simulink model "Pruning_observer_inexact"  (R2019b)
settings: Solver=VariableStepAuto  StartTime=0.0  StopTime=20  RelTol=1e-3
values from neighbouring files (symbols this model uses):
  d = 0.1    [Dynamicfcn.m]    (also in Run_this_file_for_DDWMR_model.m; gps.m)
  eta = 0.8    [Run_this_file_for_DDWMR_model.m]
  I = 0.05    [Dynamicfcn.m]    (also in Run_this_file_for_DDWMR_model.m = 0.26903125)
  L = 0.235/2    (= 0.1175)    [Dynamicfcn.m]    (also in Run_this_file_for_DDWMR_model.m; encoder.m)
  m = 10    [Dynamicfcn.m]    (also in Run_this_file_for_DDWMR_model.m = 15)
  q_initial = [theta_0;x_0;y_0]    [Run_this_file_for_DDWMR_model.m]
  r = 0.05    [Dynamicfcn.m]    (also in Run_this_file_for_DDWMR_model.m; encoder.m; robustness_support.m = temp_r(N+1:-1:1))
  R = 1e-3    (= 0.001)    [Run_this_file_for_DDWMR_model.m]
  rp = 0.6    [Run_this_file_for_DDWMR_model.m]
  s = 0.5    [Run_this_file_for_DDWMR_model.m]    (also in robustness_support.m = -(1-p)./p)
  Ts = 0.01    [Dynamicfcn.m]    (also in Run_this_file_for_DDWMR_model.m; gps.m = 0.001)
  V_initial = [v_0;w_0]    [Run_this_file_for_DDWMR_model.m]
libraries: simulink x3, sharedTrackingLibrary x1
settings Model: Creator=yu zheng  LastModifiedBy=yu zheng
settings DataIOCC: ReturnWorkspaceOutputsName=out_pruning

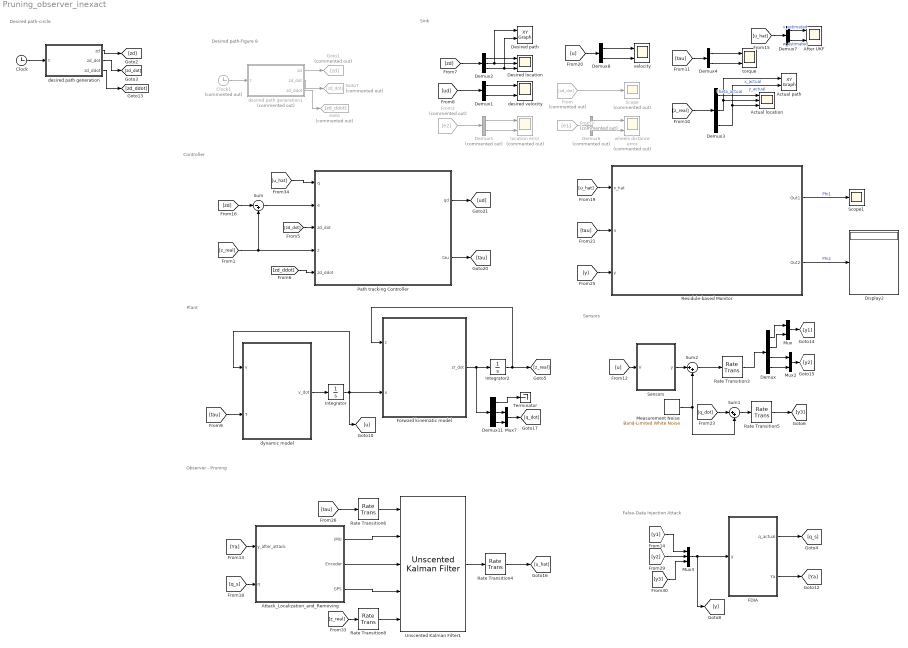
== system Pruning_observer_inexact ==
  note: Sink
  note: Controller
  note: Observer - Pruning
  note: Sensors
  note: Plant
  note: False-Data Injection Attack
  note: Desired path-circle
  note: Desired path-figure 8
  Actual location : Scope  NumInputPorts=3
  Actual path : simulink/Sinks/XY Graph  xmin=-2  xmax=2  ymin=-2  ymax=2  st=-1
  After UKF : Scope  NumInputPorts=2
  Attack_Localization_and_Removing : Subsystem
  Clock : Clock
  Clock1 : Clock  Commented=on
  Demux : Demux
  Demux{1,4,7..8} (4 alike) : Demux  Outputs=2
  Demux11 : Demux  Outputs=3
  Demux2 : Demux  Outputs=3
  Demux3 : Demux  Outputs=3
  Demux5 : Demux  Commented=on  Outputs=2
  Demux6 : Demux  Commented=on  Outputs=2
  Desired location : Scope  NumInputPorts=3
  "Desired path " : simulink/Sinks/XY Graph  xmin=-2  xmax=2  ymin=-2  ymax=2  st=-1
  Display2 : Display
  FDIA : MATLAB Function  TreatAsAtomicUnit=on
  Forward kinematic model : MATLAB Function  TreatAsAtomicUnit=on
  From : From  Commented=on  GotoTag=ud_dot
  From2 : From  Commented=on  GotoTag=e2
  From3 : From  Commented=on  GotoTag=e1
  Goto : Goto  Commented=on  GotoTag=zd_ddot
  Goto1 : Goto  Commented=on  GotoTag=zd
  Goto7 : Goto  Commented=on  GotoTag=zd_dot
  Integrator : Integrator  InitialCondition=V_initial
  Integrator2 : Integrator  InitialCondition=q_initial
  Measurement Noise : simulink/Sources/Band-Limited White Noise  Cov=R*Ts  Ts=Ts  seed=[23341]
  Mux : Mux  Inputs=2
  Mux2 : Mux  Inputs=2
  Mux3 : Mux  Inputs=3
  Mux7 : Mux  Inputs=2
  Path tracking Controller : MATLAB Function  TreatAsAtomicUnit=on
  Rate Transition3 : RateTransition  InitialCondition=[0 0 0 0]  OutPortSampleTime=Ts
  Rate Transition4 : RateTransition  Integrity=off  InitialCondition=1.6  OutPortSampleTime=0
  Rate Transition5 : RateTransition  InitialCondition=[0 0 ]  OutPortSampleTime=Ts
  Rate Transition6 : RateTransition  InitialCondition=[0 0]  OutPortSampleTime=Ts
  Rate Transition8 : RateTransition  InitialCondition=[0 0 0]  OutPortSampleTime=Ts
  Residule-based Monitor : Subsystem
  Scope : Scope  Commented=on
  Scope1 : Scope
  Sensors : MATLAB Function  TreatAsAtomicUnit=on
  Sum : Sum  Inputs=|-+
  Sum1 : Sum  Inputs=|++
  Sum2 : Sum  Inputs=|++
  Terminator : Terminator
  Unscented Kalman Filter1 : sharedTrackingLibrary/Unscented Kalman Filter  StateTransitionFcn=Dynamicfcn  HasAdditiveProcessNoise=Additive  ProcessNoise=diag([1 1])  HasTimeVaryingProcessNoise=off  HasStateTransitionFcnExtraArgument=1  InitialState=[0 0]  InitialStateCovariance=1e-2  Alpha=1e-2  Beta=2  Kappa=0  MeasurementFcn1=gyroscope  HasMeasurementEnablePort1=off  HasAdditiveMeasurementNoise1=Additive  MeasurementNoise1=diag([R R])  HasTimeVaryingMeasurementNoise1=off  HasMeasurementFcnExtraArgument1=0  MeasurementFcn2=encoder  HasMeasurementEnablePort2=off  HasAdditiveMeasurementNoise2=Additive  MeasurementNoise2=diag([R R])  HasTimeVaryingMeasurementNoise2=off  HasMeasurementFcnExtraArgument2=0  MeasurementFcn3=gps  HasMeasurementEnablePort3=off  HasAdditiveMeasurementNoise3=Additive  MeasurementNoise3=diag([R R])  HasTimeVaryingMeasurementNoise3=off  HasMeasurementFcnExtraArgument3=1  MeasurementFcn4=mfcn3  HasMeasurementEnablePort4=off  HasAdditiveMeasurementNoise4=Additive  MeasurementNoise4=R  HasTimeVaryingMeasurementNoise4=off  HasMeasurementFcnExtraArgument4=0  MeasurementFcn5=myMeasurementFcn  HasMeasurementEnablePort5=off  HasAdditiveMeasurementNoise5=Additive  MeasurementNoise5=1  HasTimeVaryingMeasurementNoise5=off  HasMeasurementFcnExtraArgument5=0  EnableMultirate=off  StateTransitionFcnSampleTime=1  MeasurementFcn1SampleTime=1  MeasurementFcn2SampleTime=1  MeasurementFcn3SampleTime=1  MeasurementFcn4SampleTime=1  MeasurementFcn5SampleTime=1  UseCurrentEstimator=on  OutputStateCovariance=off  DataType=double  SampleTime=Ts  NumberOfMeasurements=3
      settings: SourceProductName=Automated Driving Toolbox  SourceProductBaseCode=DR
  desired path generation : MATLAB Function  TreatAsAtomicUnit=on
  desired path generation1 : MATLAB Function  Commented=on  TreatAsAtomicUnit=on
  desired velocity : Scope  NumInputPorts=2
  dynamic model : MATLAB Function  TreatAsAtomicUnit=on
  location error : Scope  Commented=on  NumInputPorts=2
  torque : Scope  NumInputPorts=2
  velocity : Scope  NumInputPorts=2
  wheels distance error : Scope  Commented=on  NumInputPorts=2
  wires:
  Demux3/2 -> Actual path/1, Actual location/2  "x_actual"
  Demux/1 -> Mux/1
  Demux11/1 -> Terminator/1
  Demux3/3 -> Actual path/2, Actual location/3  "y_actual"
  Unscented Kalman Filter1/1 -> Rate Transition4/1
  From/1 -> Scope/1
  Demux/4 -> Mux2/2
  Demux1/1 -> desired velocity/1
  Demux2/1 -> Desired location/1
  Demux1/2 -> desired velocity/2
  [tau] -> dynamic model/2(T)
  [q_dot] -> Sum1/1
  Demux6/2 -> wheels distance error/2
  Demux6/1 -> wheels distance error/1
  Demux7/1 -> After UKF/1  "v_estimated"
  [tau] -> Demux4/1
  [zd] -> Demux2/1
  [ud] -> Demux1/1
  Demux11/2 -> Mux7/1
  [u_hat] -> Demux7/1
  Demux4/1 -> torque/1
  Rate Transition5/1 -> [y3]
  Demux7/2 -> After UKF/2  "w_estimated"
  Demux/3 -> Mux2/1
  [u] -> Demux8/1
  Mux/1 -> [y1]
  Demux3/1 -> Actual location/1  "theta_actual"
  Demux4/2 -> torque/2
  Demux5/1 -> location error/1
  Mux2/1 -> [y2]
  Rate Transition6/1 -> Unscented Kalman Filter1/1
  [z_real] -> Demux3/1
  From2/1 -> Demux5/1
  Forward kinematic model/1(zr_dot) -> Demux11/1, Integrator2/1
  Demux11/3 -> Mux7/2
  Sensors/1(y) -> Sum2/1
  Sum1/1 -> Rate Transition5/1
  Rate Transition8/1 -> Unscented Kalman Filter1/5
  Integrator2/1 -> [z_real], Forward kinematic model/1(z)
  Demux/2 -> Mux/2
  Mux7/1 -> [q_dot]
  Demux2/3 -> "Desired path "/2, Desired location/3
  [u] -> Sensors/1(V)
  Integrator/1 -> Forward kinematic model/2(u), dynamic model/1(v), [u]
  dynamic model/1(v_dot) -> Integrator/1
  Measurement Noise/1 -> Sum1/2, Sum2/2
  Demux5/2 -> location error/2
  Demux8/2 -> velocity/2
  [tau] -> Rate Transition6/1
  Rate Transition4/1 -> [u_hat]
  Demux2/2 -> "Desired path "/1, Desired location/2
  Demux8/1 -> velocity/1
  From3/1 -> Demux6/1
  [z_real] -> Rate Transition8/1
  Sum2/1 -> Rate Transition3/1
  Rate Transition3/1 -> Demux/1
  [q_s] -> Attack_Localization_and_Removing/2(q)
  [Ya] -> Attack_Localization_and_Removing/1(y_after_attack)
  Attack_Localization_and_Removing/3(GPS) -> Unscented Kalman Filter1/4
  Attack_Localization_and_Removing/2(Encoder) -> Unscented Kalman Filter1/3
  Attack_Localization_and_Removing/1(IMU) -> Unscented Kalman Filter1/2
  FDIA/2(Ya) -> [Ya]
  Mux3/1 -> [y], FDIA/1(y)
  [y3] -> Mux3/3
  [y1] -> Mux3/1
  [y2] -> Mux3/2
  FDIA/1(q_actual) -> [q_s]
  [u_hat] -> Residule-based Monitor/1(x_hat)
  Residule-based Monitor/2(Out2) -> Display2/1  "Phi2"
  Residule-based Monitor/1(Out1) -> Scope1/1  "Phi1"
  [tau] -> Residule-based Monitor/2(u)
  [y] -> Residule-based Monitor/3(y)
  [u_hat] -> Path tracking Controller/1(q)
  [zd_ddot] -> Path tracking Controller/5(zd_ddot)
  Sum/1 -> Path tracking Controller/2(e)
  [zd_dot] -> Path tracking Controller/3(zd_dot)
  [zd] -> Sum/1
  [z_real] -> Sum/2, Path tracking Controller/4(z)
  Path tracking Controller/1(qd) -> [ud]
  Path tracking Controller/2(tau) -> [tau]
  desired path generation/3(zd_ddot) -> [zd_ddot]
  Clock/1 -> desired path generation/1(t)
  desired path generation/1(zd) -> [zd]
  desired path generation/2(zd_dot) -> [zd_dot]
  desired path generation1/3(zd_ddot) -> Goto/1
  Clock1/1 -> desired path generation1/1(t)
  desired path generation1/1(zd) -> Goto1/1
  desired path generation1/2(zd_dot) -> Goto7/1

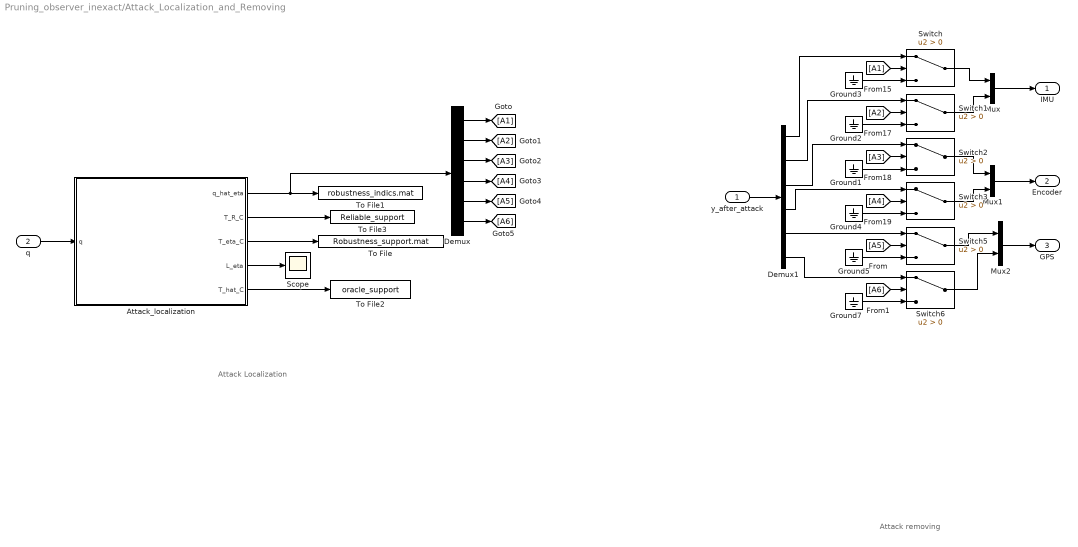
== system Pruning_observer_inexact/Attack_Localization_and_Removing ==
  note: Attack removing
  note: Attack Localization
  y_after_attack : Inport
  q : Inport  Port=2
  Attack_localization : MATLAB Function  TreatAsAtomicUnit=on
  Demux : Demux  Outputs=6
  Demux1 : Demux  Outputs=6
  Ground{1..5,7} (6 alike) : Ground
  Mux : Mux  Inputs=2
  Mux1 : Mux  Inputs=2
  Mux2 : Mux  Inputs=2
  Scope : Scope
  Switch{,1..3,5..6} (6 alike) : Switch  Criteria=u2 > Threshold
  To File : ToFile  Filename=Robustness_support.mat  MatrixName=T_eta
  To File1 : ToFile  Filename=robustness_indics.mat  MatrixName=q_hat_eta
  To File2 : ToFile  Filename=oracle_support  MatrixName=T_hat
  To File3 : ToFile  Filename=Reliable_support  MatrixName=T_R
  IMU : Outport
  Encoder : Outport  Port=2
  GPS : Outport  Port=3
  wires:
  Attack_localization/4(L_eta) -> Scope/1
  Attack_localization/2(T_R_C) -> To File3/1
  Attack_localization/5(T_hat_C) -> To File2/1
  Attack_localization/3(T_eta_C) -> To File/1
  [A3] -> Switch2/2
  [A4] -> Switch3/2
  [A2] -> Switch1/2
  [A1] -> Switch/2
  Switch/1 -> Mux/1
  Switch1/1 -> Mux/2
  Switch2/1 -> Mux1/1
  Switch3/1 -> Mux1/2
  Switch6/1 -> Mux2/2
  Attack_localization/1(q_hat_eta) -> Demux/1, To File1/1
  Demux/1 -> [A1]
  Demux/2 -> [A2]
  Demux/3 -> [A3]
  Demux/4 -> [A4]
  Demux/5 -> [A5]
  Demux/6 -> [A6]
  y_after_attack/1 -> Demux1/1
  Mux/1 -> IMU/1
  Mux2/1 -> GPS/1
  q/1 -> Attack_localization/1(q)
  Ground3/1 -> Switch/3
  Demux1/1 -> Switch/1
  Ground2/1 -> Switch1/3
  Ground1/1 -> Switch2/3
  Ground4/1 -> Switch3/3
  Ground5/1 -> Switch5/3
  Ground7/1 -> Switch6/3
  Demux1/2 -> Switch1/1
  Demux1/3 -> Switch2/1
  Demux1/4 -> Switch3/1
  Demux1/5 -> Switch5/1
  Demux1/6 -> Switch6/1
  [A5] -> Switch5/2
  [A6] -> Switch6/2
  Mux1/1 -> Encoder/1
  Switch5/1 -> Mux2/1

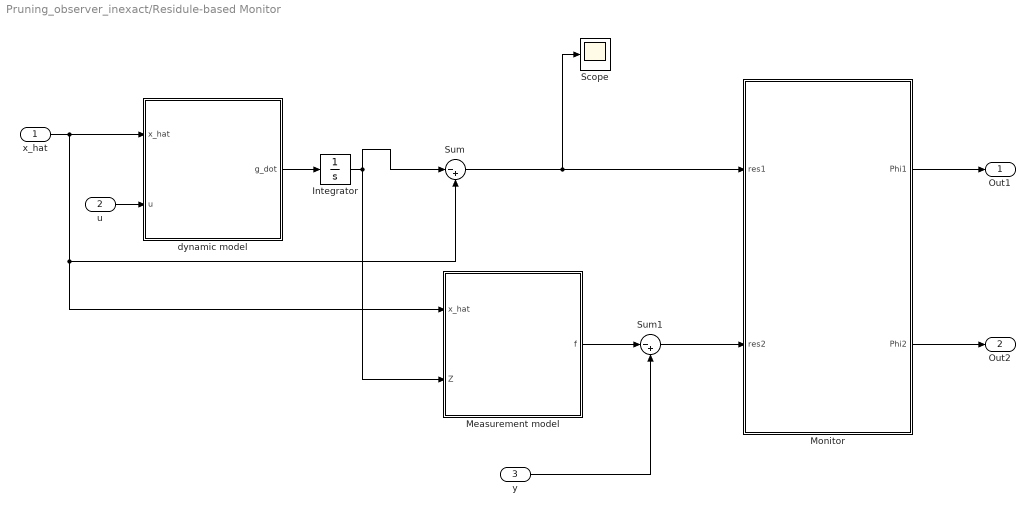
== system Pruning_observer_inexact/Residule-based Monitor ==
  x_hat : Inport
  u : Inport  Port=2
  y : Inport  Port=3
  Integrator : Integrator  InitialCondition=[0 0]
  Measurement model : MATLAB Function  TreatAsAtomicUnit=on
  Monitor : MATLAB Function  TreatAsAtomicUnit=on
  Scope : Scope
  Sum : Sum  Inputs=|-+
  Sum1 : Sum  Inputs=|-+
  dynamic model : MATLAB Function  TreatAsAtomicUnit=on
  Out1 : Outport
  Out2 : Outport  Port=2
  wires:
  dynamic model/1(g_dot) -> Integrator/1
  Integrator/1 -> Sum/1, Measurement model/2(Z)
  u/1 -> dynamic model/2(u)
  Measurement model/1(f) -> Sum1/1
  y/1 -> Sum1/2
  Sum/1 -> Scope/1, Monitor/1(res1)
  Sum1/1 -> Monitor/2(res2)
  Monitor/1(Phi1) -> Out1/1
  Monitor/2(Phi2) -> Out2/1
  x_hat/1 -> dynamic model/1(x_hat), Measurement model/1(x_hat), Sum/2

== matlab function Pruning_observer_inexact/Attack_Localization_and_Removing/Attack_localization ==
  data: q_hat_eta output; T_R_C output; q input; T_eta_C output; rp parameter; s parameter; eta parameter; L_eta output; T_hat_C output
function [q_hat_eta,T_R_C,T_eta_C,L_eta,T_hat_C] = fcn(q,rp, s, eta)
%% Obtain oracle
N=6;
[p, q_hat] = localization_oracle(q,rp);
T_hat_CTemp = find(q_hat);
T_hat_C = zeros(N,1);
T_hat_C(1:size(T_hat_CTemp,1))=T_hat_CTemp(1:size(T_hat_CTemp,1));    % constraint the decimation of the estimated support vector

%% Obtain robustness support
[R_idx_C,T_hat_eta_C,q_hat_eta,L_eta] = robustness_support(p,T_hat_CTemp,s,eta);
T_eta_C = zeros(N,1);              % maintain the size of vector of support is constant (for simulation in simulink)
if isempty(T_hat_eta_C)
    T_eta_C = zeros(N,1); 
else
    T_eta_C(1:size(T_hat_eta_C,1))=T_hat_eta_C(1:size(T_hat_eta_C,1));
end
T_R_C = zeros(N,1);             
if isempty(R_idx_C)
    T_R_C = zeros(N,1); 
else
    T_R_C(1:size(R_idx_C,1))=R_idx_C(1:size(R_idx_C,1));
end

end

== matlab function Pruning_observer_inexact/Residule-based Monitor/dynamic model ==
  data: x_hat input; g_dot output; u input; m parameter; d parameter; I parameter; L parameter; r parameter
function g_dot = fcn(x_hat,u,m, d, I, L, r)
omega=x_hat(2);

M_temp=[m*d*d+I,0;
         0,m];

M_inver=(1/(m*(m*d*d+I)))*M_temp;

D=[0,-m*d*omega;
    m*d*omega,0];

B=(1/r)*[1,1;L,-L];

g_dot=M_inver*(-D*x_hat+B*u);

== matlab function Pruning_observer_inexact/FDIA ==
  data: q_actual output; y input; Ya output; d parameter; r parameter; L parameter; Ts parameter; m parameter; I parameter
function [q_actual,Ya] = fcn(y,d,r, L, Ts, m, I)

%% Obtain coding matrix for each time step
theta0=pi/2;
v0=1;
omega0=1;
n  = 3;
T  = 6;    % time horizon (set it equal to number of measurements)

M = diag([m, m*d^2+I]);
D = [0 m*d*omega0;m*d*omega0 0];

C = [                  0,                       1,            0;
                        0,                       0,            1;
                        0,                      1/(4*r),     L/(4*r);
                        0,                      1/(4*r),     -L/(4*r); 
      -v0*sin(theta0)-d*omega0*cos(theta0),  cos(theta0), -d*sin(theta0);
       v0*cos(theta0)+d*omega0*sin(theta0),  sin(theta0),  d*cos(theta0)];
 Cd = C;
 
%  A = [   0,           0,                       1;
%          0,           0,                  2*d*omega0;
%          0,    -m*d*omega0/(m*d^2+I),    -m*d*v0/(m*d^2+I) ];

A = [0 0 1;
     zeros(2,1) -inv(M)*D];

N = size(Cd,1);
Ad = eye(n)+Ts*A;
H = zeros(N*(T+1),n);
%  ya = zeros(N*(T+1),1);
 
 
%% Actual test

% random process to decide the attack nodes
p = 0.8;  % attack (1-p) percentage e.g 20% measurement nodes is attacked
n_safe = fix(p*N); % number of safe measurements
n_attack = N-n_safe; % number of attacked channels

[I_attack_local] = getAttackIndices(Cd,n_attack);

% I_attack = zeros(n_attack*(T+1),1);

% FDIA generation parameters
max_attack = 500;  % maximum allowable attack
tau = .1;   % escape parameter for BDD
I_attack = zeros(n_attack*(T+1),1);
for index=1:(T+1)
    % Building measurement model (linearized)
    H(((index-1)*N+1):(index*N),:) = Cd*Ad^(index-1);  % measurment matrix

    % generating attack indices
%     q = zeros(N,1);
%     q(randperm(N,n_safe)) = 1;
%     I_attack_local = find(~q);  % the attck indices at the current time

    I_attack(((index-1)*n_attack+1):(index*n_attack)) = (index-1)*N + I_attack_local;
        
%     ya(((index-1)*N+1):(index*N),1) = gen_attack_channel(H(((index-1)*size(C,1)+1):(index*size(C,1)),:), max_attack,I_attack,tau);
    
end

ya = gen_attack_channel(H,max_attack,I_attack,tau);

Ya = y+ya(1:N);

q_actual = zeros(6,1);
for ii=1:N
    if ya(ii) == 0
    q_actual(ii) = 1;
    end
end

== matlab function Pruning_observer_inexact/Sensors ==
  data: V input; y output; r parameter; L parameter
function y = fcn(V,r,L)

C=[1,0;
    0,1;
    1/(4*r),L/(4*r);
    1/(4*r),-L/(4*r)];
y=C*V;

== matlab function Pruning_observer_inexact/Path tracking Controller ==
  data: qd output; q input; tau output; e input; zd_dot input; z input; zd_ddot input; m parameter; d parameter; r parameter; L parameter; I parameter
function [qd,tau] = fcn(q,e,zd_dot,z,zd_ddot,m, d, r, L, I)


kq =15;
ke =15;
ez = e(2:3);
% e_theta = e(1);
theta = z(1);
omega = q(2);

B_inver=-(r/(2*L))*[-L,-1;-L,1];
M=[m,0;
    0,m*d*d+I];
D=[0,-m*d*omega;
    m*d*omega,0];
C = [cos(theta), -d*sin(theta);
     sin(theta), d*cos(theta)];
C_bar_tran = [0, cos(theta), sin(theta);
              1, -d*sin(theta), d*cos(theta)];
C_inver = (1/d)*[d*cos(theta), d*sin(theta);
                 -sin(theta), cos(theta)];
C_inver_dot = (1/d)*[-d*sin(theta)*omega, d*cos(theta)*omega;
                     -cos(theta)*omega, -sin(theta)*omega];


qd = C_inver*(zd_dot-ke*ez);
qd_dot = -ke*(C_inver_dot*ez+q)+C_inver*(zd_ddot+ke*zd_dot+C*C_inver_dot*zd_dot);
u = -kq*(q-qd)+qd_dot-C_bar_tran*e;
tau = B_inver*(M*u+D*q);

== matlab function Pruning_observer_inexact/desired path generation1 ==
  data: t input; zd output; zd_dot output; zd_ddot output
function [zd,zd_dot,zd_ddot] = fcn(t)

a=1;
x = a*cos(t)/(1+sin(t)^2);
y = a*sin(t)*cos(t)/(1+sin(t)^2);
% unit circle (radius = 1; origin: (0,0))
zd = [atan(y./x);              % theta
      a*cos(t)/(1+sin(t)^2);         % x
      a*sin(t)*cos(t)/(1+sin(t)^2)];        % y

zd_dot = [-a*sin(t)*(cos(t)^2+2)/(1+sin(t)^2)^2;
          (a*cos(t)^2-2*a*sin(t)^2)/(1+sin(t)^2)^2];

z1 = (a*sin(t)^2*cos(t)^3-11*a*cos(t)^3+8*a*cos(t))/(1+sin(t)^2)^3;
z2 = -2*a*sin(t)*cos(t)*(3+2*cos(t)^2-sin(t)^2)/(1+sin(t)^2)^3;
zd_ddot = [z1;
           z2];

== matlab function Pruning_observer_inexact/Residule-based Monitor/Measurement model ==
  data: x_hat input; f output; Z input; L parameter; r parameter; d parameter
function f = fcn(x_hat,Z,L, r, d)
theta = Z(1);
C=[1,0;
    0,1;
    1/(4*r),L/(4*r);
    1/(4*r),-L/(4*r);
    cos(theta), -d*sin(theta);
    sin(theta), d*cos(theta)  ];
f=C*x_hat;

== matlab function Pruning_observer_inexact/Residule-based Monitor/Monitor ==
  data: res1 input; res2 input; Phi1 output; Phi2 output
function [Phi1,Phi2] = fcn(res1,res2)
%%
% is a residual-based monitor on T time-horizon.
%
% Inputs: 
%     - res1: x_hat_{j+1}-g(x_hat_j,u-j)
%     - res2: y_j - f(x_hat_j)
% Outputs:
%     - Phi1: 0(safe), 1(unsafe)
%     - Phi2: support of attack location
% Parameters:


N = size(res2,1);
n = size(res1,1);
T = N+1;

%% monitor scheme
%
% Idea: At each time step, test for every state and measurement.
%       output1 (0:safe, 1:unsafe): use a (N+n)-by-T to disaplay every
%       state and measurement testing result
%       output2 (2^[N-by-1]): give the location support of attack
%                             if at one time, one node is identified as
%                             attacked, the corresponding elements keep as
%                             attacked
epsilon_v = 15;
epsilon_w = 15;

phi1 = zeros(N+n,T);
Phi2 = ones(N,1);

for indexT = 1:T
    for index1 = 1:N
    if abs(norm(res2(index1))) > epsilon_w
        phi1(index1,indexT) = 1;
        Phi2(index1) = 2^index1;
    else
        phi1(index1,indexT) = 0;
        if Phi2(index1) == 1
            Phi2(index1) = 2^0;
        end
    end
    end
    for index2 = 1:n
    if abs(norm(res1(index2))) > epsilon_v
        phi1(N+index2,indexT) = 1;
    else
        phi1(N+index2,indexT) = 0;
    end
    end
end
if norm(phi1,1) ~=0
    Phi1 = 1;
else
    Phi1 = 0;
end
end

== matlab function Pruning_observer_inexact/Forward kinematic model ==
  data: z input; u input; zr_dot output; d parameter; r parameter
function zr_dot = fcn(z,u,d,r)

%% unpacking the state vectors
theta=z(1);

%% unpacking the intput
v=u(1);
omega=u(2);

%% ODE
theta_dot=omega;
x_dot=v*cos(theta)-d*omega*sin(theta);
y_dot=v*sin(theta)+d*omega*cos(theta);
% phir_dot = (v+omega)/r;
% phil_dot = (v-omega)/r;


%% packing the output
zr_dot=[theta_dot;x_dot;y_dot];

== matlab function Pruning_observer_inexact/dynamic model ==
  data: v_dot output; v input; T input; L parameter; r parameter; d parameter; m parameter; I parameter
function v_dot = fcn(v, T,L, r, d, m,I)

%% unpacking intput
omega=v(2);

%% Parameter
M_temp=[m*d*d+I,0;
         0,m];

M_inver=(1/(m*(m*d*d+I)))*M_temp;

D=[0,-m*d*omega;
    m*d*omega,0];

B=(1/r)*[1,1;L,-L];

%% ODE
v_dot=M_inver*(-D*v+B*T);

== matlab function Pruning_observer_inexact/desired path generation ==
  data: t input; zd output; zd_dot output; zd_ddot output
function [zd,zd_dot,zd_ddot] = fcn(t)


% unit circle (radius = 1; origin: (0,0))
zd = [t;
      cos(t);         % x
      sin(t)];        % y

zd_dot = [-sin(t);
          cos(t)];
      
zd_ddot = [-cos(t);
           -sin(t)];
